simulink model "new_nncACCsystem_4_50"  (R2021a)
(part 10 of 11)

  "IW{4,3}(50,:)'" : Constant  Value=[-0.68975039419682138142064786734408698976039886474609375;-0.337703855474782710377468220031005330383777618408203125;-0.221193087362799634121302005951292812824249267578125;-0.413240348725000650187411110891844145953655242919921875;0.7056367750395093896287335155648179352283477783203125;-0.8247240414571177513636257572215981781482696533203125;-0.368456059408796943177577531969291158020496368408203125;-0.1846558397734467948936298853368498384952545166015625;0.0934305421607941610773195861838757991790771484375;-0.034656334463735671835848961563897319138050079345703125;-0.0169908156708868281203894667896747705526649951934814453125;-0.2111294128865961738927836677248706109821796417236328125;-0.03301633733253335478696754989869077689945697784423828125;-0.453089555771492513702725091206957586109638214111328125;0.90942800382245103651968065605615265667438507080078125;0.784331063728789690259191047516651451587677001953125;-0.0022926906763267584921095476602204144001007080078125;-0.307120717402806775453427690081298351287841796875;0.3730766917773566948568486623116768896579742431640625;0.42980367039944067375500935668242163956165313720703125;-0.12049576378110614383043497355174622498452663421630859375;-0.4758132002910449021015892867580987513065338134765625;-0.86012741082964183636505595131893642246723175048828125;0.7717364942113531522949188001803122460842132568359375;0.4831846028324913167040222106152214109897613525390625;-0.486763294268171275991363700086367316544055938720703125;0.058798309327644800170720174037342076189815998077392578125;0.8066996306207865341519891444477252662181854248046875;-0.69255381214840194825654862142982892692089080810546875;0.1574299186005535811094802056686603464186191558837890625;-0.270336303295735158602752790102385915815830230712890625;0.055888155797568561666821551625616848468780517578125;0.94032669226065757062116290398989804089069366455078125;0.8304969527097798565051789410063065588474273681640625;0.4826285624021837694641590132960118353366851806640625;0.747021101342736582040515713742934167385101318359375;0.391904922693947888046039906839723698794841766357421875;0.764349790072494261750080113415606319904327392578125;-0.7526861421599579937691260056453756988048553466796875;0.240398710986991392957179414224810898303985595703125;-0.0888946820176654828316031853319145739078521728515625;-0.95043102468777018732026817815494723618030548095703125;0.607481136103278362980972815421409904956817626953125;0.5162479599471743174632365480647422373294830322265625;-0.6363106814400574240409014237229712307453155517578125;-0.90826116263117118165837382548488676548004150390625;0.0521855822376402489481961310957558453083038330078125;-0.35977935968636831631783934426493942737579345703125;-0.61308326456983974761527633745572529733180999755859375;-0.4875485158677352881539945883559994399547576904296875]
      mask Display: e = 0.06;c1 = [120 150 230]/255;c2 = ([120 150 230]+0)/383;c3 = ([120 150 230]+128)/383;patch([0 1 1 0],[0 0 1 1],c1);patch([0 1 1 1-e 1-e 0+e],[0 0 1 1-e 0+e 0+e],c2);patch([0 0 1 1-e 0+e 0+e],[0 1 1 1-e 1-e 0+e],c3);plot([0 1 1 0 0],[0 0 1 1 0]);disp('weights');
  "IW{4,3}(6,:)'" : Constant  Value=[0.3760934772975199624767128625535406172275543212890625;0.83188378952229680152186119812540709972381591796875;0.21646625261934016037912442698143422603607177734375;0.4175166061785808846451573117519728839397430419921875;0.245071136922079713116318089305423200130462646484375;-0.2968621138896334610279836851987056434154510498046875;-0.952473185116357701218703368795104324817657470703125;-0.2791944329040980665723736819927580654621124267578125;0.9561025717111750754639842853066511452198028564453125;-0.5509567477390866496733679014141671359539031982421875;0.191023007401977196195730357430875301361083984375;-0.6712729624144617712744320670026354491710662841796875;0.293846976010136540224948475952260196208953857421875;0.5376360375443791639327173470519483089447021484375;-0.689068301622072443279876097221858799457550048828125;-0.9420681689532297564682039592298679053783416748046875;-0.9153320513397549262890606769360601902008056640625;0.7080240151346572918811261843075044453144073486328125;-0.345534410238059308539959602057933807373046875;-0.2596236597249992339442314914776943624019622802734375;0.0156286869832829022897158210980705916881561279296875;0.8238046279287318807149631538777612149715423583984375;0.5409551194199606616308528828085400164127349853515625;-0.539752608426157909349285546340979635715484619140625;-0.47908886469649036854434598353691399097442626953125;-0.309505474526706070292902950313873589038848876953125;0.0077398428835653287904960961895994842052459716796875;-0.775756660878660131430706314858980476856231689453125;0.48844455217338822450301449862308800220489501953125;0.3564821650667175934046326801762916147708892822265625;-0.875481475304413780946788392611779272556304931640625;-0.4156409251020398709641767709399573504924774169921875;0.0110057222602060189586836713715456426143646240234375;-0.8698058882352397436221735915751196444034576416015625;0.3406812767959930265959656026097945868968963623046875;0.4584986472564220871817042279872111976146697998046875;0.5278497841276512669850262682302854955196380615234375;-0.6111457754962399402387518421164713799953460693359375;0.6732737919294760065014315841835923492908477783203125;0.33259267094354338922812530654482543468475341796875;-0.262129955270015368995473181712441146373748779296875;0.140717092303284996290813069208525121212005615234375;0.2060885085486192647152847712277434766292572021484375;-0.1796235649662640820878323211218230426311492919921875;0.4438024646861824518140338113880716264247894287109375;-0.62840596751767474614780439878813922405242919921875;0.0965023358081340543179749147384427487850189208984375;-0.056687085267606018845754078938625752925872802734375;-0.0347507703779630361395902582444250583648681640625;-0.5844728297823975626812398331821896135807037353515625]
      mask Display: e = 0.06;c1 = [120 150 230]/255;c2 = ([120 150 230]+0)/383;c3 = ([120 150 230]+128)/383;patch([0 1 1 0],[0 0 1 1],c1);patch([0 1 1 1-e 1-e 0+e],[0 0 1 1-e 0+e 0+e],c2);patch([0 0 1 1-e 0+e 0+e],[0 1 1 1-e 1-e 0+e],c3);plot([0 1 1 0 0],[0 0 1 1 0]);disp('weights');
  "IW{4,3}(7,:)'" : Constant  Value=[0.8403152974258485397029971863958053290843963623046875;-0.2071458617563731452460018545025377534329891204833984375;-0.723618348300131941641666344366967678070068359375;-0.221142697352507633379303797482862137258052825927734375;0.128396382406429532263558712656958959996700286865234375;-0.1519073900361445073059485366684384644031524658203125;0.9312006523396398893765990578685887157917022705078125;-0.1622147733336041230955970604554750025272369384765625;-0.2574608060089185190832949956529773771762847900390625;-0.7602871717810824048200402103248052299022674560546875;-0.674581332874239603114574492792598903179168701171875;0.339430166289895474118765150706167332828044891357421875;-0.051697509834940529038771472869484568946063518524169921875;0.92405403156981236190148365494678728282451629638671875;-0.85714465050820354274918599912780337035655975341796875;-0.7299230912443717134152620928944088518619537353515625;0.5437820509629733845002874659257940948009490966796875;-0.15716114414254267472870196797885000705718994140625;0.343336796613522399201912094213184900581836700439453125;0.85244575266534761137648956719203852117061614990234375;-0.366396803935940429397533080191351473331451416015625;-0.4758893825967518420583246552268974483013153076171875;-0.281940397738466297372639246532344259321689605712890625;0.25070758776880397444841719334363006055355072021484375;-0.9138567005525863873316438912297599017620086669921875;-0.97612403919302159760462700432981364428997039794921875;0.498327283343458493636290995709714479744434356689453125;0.54675754849605573415516346358344890177249908447265625;-0.81192472217370215137322020382271148264408111572265625;0.7166593175219968525624381072702817618846893310546875;-0.4585059146709802302410707852686755359172821044921875;-0.6980232397374750430429912739782594144344329833984375;-0.7518397450349640909195159110822714865207672119140625;0.973777211720303181863300778786651790142059326171875;-0.286875771908233101470386827713809907436370849609375;0.577485900634702176148493890650570392608642578125;0.3016639899357438370230966029339469969272613525390625;-0.46914794612984156430002258275635540485382080078125;0.6921957739679298615698144203634001314640045166015625;0.911826429592337728280426745186559855937957763671875;-0.097525671829564064552187119261361658573150634765625;-0.357522559522956251409908645655377767980098724365234375;-0.7465707324766157615414385873009450733661651611328125;0.8102029921478746121721314921160228550434112548828125;0.7027792710522238195380850811488926410675048828125;-0.82556198499486865838292715125135146081447601318359375;-0.5517677957555833234692954647471196949481964111328125;-0.923520812028227222612031255266629159450531005859375;0.69847535958997009064574967851513065397739410400390625;0.219645138083222446478970368843874894082546234130859375]
      mask Display: e = 0.06;c1 = [120 150 230]/255;c2 = ([120 150 230]+0)/383;c3 = ([120 150 230]+128)/383;patch([0 1 1 0],[0 0 1 1],c1);patch([0 1 1 1-e 1-e 0+e],[0 0 1 1-e 0+e 0+e],c2);patch([0 0 1 1-e 0+e 0+e],[0 1 1 1-e 1-e 0+e],c3);plot([0 1 1 0 0],[0 0 1 1 0]);disp('weights');
  "IW{4,3}(8,:)'" : Constant  Value=[-0.116688462945323312425216499832458794116973876953125;-0.44605947992465377893722688895650207996368408203125;-0.99658732093286328534986751037649810314178466796875;-0.4783079385244317638381517099332995712757110595703125;-0.2005728686337964195018912505474872887134552001953125;0.3958930317653159836055465348181314766407012939453125;0.0066115562235269376145652131526730954647064208984375;-0.12976532301678833647429200937040150165557861328125;0.862763084062491802939121043891645967960357666015625;0.7666804068579538000705042577465064823627471923828125;0.2002755332553858291788628775975666940212249755859375;0.3224981613712751826739122407161630690097808837890625;-0.7600989470280747895003514713607728481292724609375;0.71268837011036634265792599762789905071258544921875;0.2693318183489117334517004564986564218997955322265625;-0.0214151734751999445194314830587245523929595947265625;0.6479068856290701727829173250938765704631805419921875;0.9944276360022599181576197224785573780536651611328125;-0.1792349111526914118286413213354535400867462158203125;0.45674222060069258333214747835882008075714111328125;0.7704956869907266803210177386063151061534881591796875;-0.0006436272250007757378398309811018407344818115234375;-0.999483386372119309015715771238319575786590576171875;-0.85831423715791288486798293888568878173828125;0.786250856395209307692084621521644294261932373046875;-0.50744024569466983365373380365781486034393310546875;0.4816054146965200732921630333294160664081573486328125;-0.6902006291492128742248723938246257603168487548828125;0.254298316287407732971814766642637550830841064453125;0.519368061486161547435358443181030452251434326171875;-0.790785644673932086590184553642757236957550048828125;-0.68706590989727001073106293915770947933197021484375;-0.558513508754861387473056311137042939662933349609375;0.851974564750733964757500871201045811176300048828125;-0.35667622767825069018954309285618364810943603515625;-0.41145172263983109672835780656896531581878662109375;-0.6493602201676791363382790223113261163234710693359375;-0.5994916295150145568726429701200686395168304443359375;0.4041599000882392100919560107286088168621063232421875;-0.9586288357621561839749801947618834674358367919921875;-0.4832610329434474660814657909213565289974212646484375;-0.842123864413237388504285263479687273502349853515625;-0.561651447245997470503198201186023652553558349609375;0.9176915198905877257828933579730801284313201904296875;-0.43094663445379222110886985319666564464569091796875;0.714815990308057536140040610916912555694580078125;-0.1655937814369423666249758753110654652118682861328125;0.4845374606734373923444536558235995471477508544921875;0.24719870091719453597534084110520780086517333984375;-0.1506864718307741046743331025936640799045562744140625]
      mask Display: e = 0.06;c1 = [120 150 230]/255;c2 = ([120 150 230]+0)/383;c3 = ([120 150 230]+128)/383;patch([0 1 1 0],[0 0 1 1],c1);patch([0 1 1 1-e 1-e 0+e],[0 0 1 1-e 0+e 0+e],c2);patch([0 0 1 1-e 0+e 0+e],[0 1 1 1-e 1-e 0+e],c3);plot([0 1 1 0 0],[0 0 1 1 0]);disp('weights');
  "IW{4,3}(9,:)'" : Constant  Value=[0.954560714917990882355525172897614538669586181640625;0.3907355247891455274356076188269071280956268310546875;0.4785140467488202542511999126872979104518890380859375;-0.376592379022518797260232759072096087038516998291015625;0.893300544264355789181308864499442279338836669921875;-0.193749178232689001077915236237458884716033935546875;-0.46602024758462778919465563376434147357940673828125;-0.2137706950459603572056721532135270535945892333984375;-0.295088615243286778166975636850111186504364013671875;-0.55059251882629689500703307203366421163082122802734375;0.1859857246918747986086373202851973474025726318359375;-0.7383847097081759347503293611225672066211700439453125;0.95986875357167089628518397148582153022289276123046875;-0.54077786815700668032746989410952664911746978759765625;-0.9628262032856012009318646960309706628322601318359375;0.59317539902114280181422145687974989414215087890625;0.58436536663263805024826069711707532405853271484375;-0.5340179474788222524495040488545782864093780517578125;0.75937146836898661295123247327865101397037506103515625;-0.676442785071257102202935129753313958644866943359375;-0.855504824920894524353798260563053190708160400390625;-0.13403199832274792502317950493306852877140045166015625;-0.110797775178757884617652962333522737026214599609375;-0.051205157018530782220278041450001182965934276580810546875;-0.1871836746140778107161395382718183100223541259765625;-0.140905405881837142434420684367069043219089508056640625;-0.783364454271953558617269663955084979534149169921875;0.2111641315298364018904209160609752871096134185791015625;0.910823829267612961047007047454826533794403076171875;0.231589466193370230318038238692679442465305328369140625;0.310157527484731632139158818972646258771419525146484375;0.4978665952885050760556850946159102022647857666015625;-0.387506558926215216587252143654040992259979248046875;0.96150365795292291881679602738586254417896270751953125;-0.094735304889166815911494268220849335193634033203125;0.967857219447221250874235920491628348827362060546875;-0.2322423485804778753305299687781371176242828369140625;0.74864662580344454312353263958357274532318115234375;0.9489155620308868943624247549450956284999847412109375;-0.4060423979950436024211057883803732693195343017578125;0.3119893689463706376585605539730750024318695068359375;0.1879491277425034134740400304508511908352375030517578125;0.93771791705965490404395268342341296374797821044921875;0.4005764539610321417484328776481561362743377685546875;0.35793568702171862927485790351056493818759918212890625;-0.710784392004865761549581293365918099880218505859375;-0.349110480398596489948204180109314620494842529296875;0.0559771506617912084635690916911698877811431884765625;0.07350224902426032158597735133298556320369243621826171875;-0.50203355681308015068253780555096454918384552001953125]
      mask Display: e = 0.06;c1 = [120 150 230]/255;c2 = ([120 150 230]+0)/383;c3 = ([120 150 230]+128)/383;patch([0 1 1 0],[0 0 1 1],c1);patch([0 1 1 1-e 1-e 0+e],[0 0 1 1-e 0+e 0+e],c2);patch([0 0 1 1-e 0+e 0+e],[0 1 1 1-e 1-e 0+e],c3);plot([0 1 1 0 0],[0 0 1 1 0]);disp('weights');
  Mux : Mux  Inputs=50
      mask Display: e = 0.06;c1 = [120 150 230]/255;c2 = ([120 150 230]+0)/383;c3 = ([120 150 230]+128)/383;patch([0 1 1 0],[0 0 1 1],c1);patch([0 1 1 1-e 1-e 0+e],[0 0 1 1-e 0+e 0+e],c2);patch([0 0 1 1-e 0+e 0+e],[0 1 1 1-e 1-e 0+e],c3);plot([0 1 1 0 0],[0 0 1 1 0]);disp('Mux');
  dotprod{1..50} (50 alike) : neural/Weight Functions/dotprod
  "lz{4,3}" : Outport
      mask Display: e = 0.06;c1 = [120 230 180]/255;c2 = ([120 230 180]+0)/(256+128);c3 = ([120 230 180]+128)/(256+128);patch([0 1 1 0],[0 0 1 1],c1);patch([0 1 1 1-e 1-e 0+e],[0 0 1 1-e 0+e 0+e],c2);patch([0 0 1 1-e 0+e 0+e],[0 1 1 1-e 1-e 0+e],c3);plot([0 1 1 0 0],[0 0 1 1 0]);
  wires:
  "IW{4,3}(1,:)'"/1 -> dotprod1/1
  "ad{4,3}"/1 -> dotprod1/2, dotprod2/2, dotprod3/2, dotprod4/2, dotprod5/2, dotprod6/2, dotprod7/2, dotprod8/2, dotprod9/2, dotprod10/2, dotprod11/2, dotprod12/2, dotprod13/2, dotprod14/2, dotprod15/2, dotprod16/2, dotprod17/2, dotprod18/2, dotprod19/2, dotprod20/2, dotprod21/2, dotprod22/2, dotprod23/2, dotprod24/2, dotprod25/2, dotprod26/2, dotprod27/2, dotprod28/2, dotprod29/2, dotprod30/2, dotprod31/2, dotprod32/2, dotprod33/2, dotprod34/2, dotprod35/2, dotprod36/2, dotprod37/2, dotprod38/2, dotprod39/2, dotprod40/2, dotprod41/2, dotprod42/2, dotprod43/2, dotprod44/2, dotprod45/2, dotprod46/2, dotprod47/2, dotprod48/2, dotprod49/2, dotprod50/2
  dotprod1/1 -> Mux/1
  "IW{4,3}(2,:)'"/1 -> dotprod2/1
  dotprod2/1 -> Mux/2
  "IW{4,3}(3,:)'"/1 -> dotprod3/1
  dotprod3/1 -> Mux/3
  "IW{4,3}(4,:)'"/1 -> dotprod4/1
  dotprod4/1 -> Mux/4
  "IW{4,3}(5,:)'"/1 -> dotprod5/1
  dotprod5/1 -> Mux/5
  "IW{4,3}(6,:)'"/1 -> dotprod6/1
  dotprod6/1 -> Mux/6
  "IW{4,3}(7,:)'"/1 -> dotprod7/1
  dotprod7/1 -> Mux/7
  "IW{4,3}(8,:)'"/1 -> dotprod8/1
  dotprod8/1 -> Mux/8
  "IW{4,3}(9,:)'"/1 -> dotprod9/1
  dotprod9/1 -> Mux/9
  "IW{4,3}(10,:)'"/1 -> dotprod10/1
  dotprod10/1 -> Mux/10
  "IW{4,3}(11,:)'"/1 -> dotprod11/1
  dotprod11/1 -> Mux/11
  "IW{4,3}(12,:)'"/1 -> dotprod12/1
  dotprod12/1 -> Mux/12
  "IW{4,3}(13,:)'"/1 -> dotprod13/1
  dotprod13/1 -> Mux/13
  "IW{4,3}(14,:)'"/1 -> dotprod14/1
  dotprod14/1 -> Mux/14
  "IW{4,3}(15,:)'"/1 -> dotprod15/1
  dotprod15/1 -> Mux/15
  "IW{4,3}(16,:)'"/1 -> dotprod16/1
  dotprod16/1 -> Mux/16
  "IW{4,3}(17,:)'"/1 -> dotprod17/1
  dotprod17/1 -> Mux/17
  "IW{4,3}(18,:)'"/1 -> dotprod18/1
  dotprod18/1 -> Mux/18
  "IW{4,3}(19,:)'"/1 -> dotprod19/1
  dotprod19/1 -> Mux/19
  "IW{4,3}(20,:)'"/1 -> dotprod20/1
  dotprod20/1 -> Mux/20
  "IW{4,3}(21,:)'"/1 -> dotprod21/1
  dotprod21/1 -> Mux/21
  "IW{4,3}(22,:)'"/1 -> dotprod22/1
  dotprod22/1 -> Mux/22
  "IW{4,3}(23,:)'"/1 -> dotprod23/1
  dotprod23/1 -> Mux/23
  "IW{4,3}(24,:)'"/1 -> dotprod24/1
  dotprod24/1 -> Mux/24
  "IW{4,3}(25,:)'"/1 -> dotprod25/1
  dotprod25/1 -> Mux/25
  "IW{4,3}(26,:)'"/1 -> dotprod26/1
  dotprod26/1 -> Mux/26
  "IW{4,3}(27,:)'"/1 -> dotprod27/1
  dotprod27/1 -> Mux/27
  "IW{4,3}(28,:)'"/1 -> dotprod28/1
  dotprod28/1 -> Mux/28
  "IW{4,3}(29,:)'"/1 -> dotprod29/1
  dotprod29/1 -> Mux/29
  "IW{4,3}(30,:)'"/1 -> dotprod30/1
  dotprod30/1 -> Mux/30
  "IW{4,3}(31,:)'"/1 -> dotprod31/1
  dotprod31/1 -> Mux/31
  "IW{4,3}(32,:)'"/1 -> dotprod32/1
  dotprod32/1 -> Mux/32
  "IW{4,3}(33,:)'"/1 -> dotprod33/1
  dotprod33/1 -> Mux/33
  "IW{4,3}(34,:)'"/1 -> dotprod34/1
  dotprod34/1 -> Mux/34
  "IW{4,3}(35,:)'"/1 -> dotprod35/1
  dotprod35/1 -> Mux/35
  "IW{4,3}(36,:)'"/1 -> dotprod36/1
  dotprod36/1 -> Mux/36
  "IW{4,3}(37,:)'"/1 -> dotprod37/1
  dotprod37/1 -> Mux/37
  "IW{4,3}(38,:)'"/1 -> dotprod38/1
  dotprod38/1 -> Mux/38
  "IW{4,3}(39,:)'"/1 -> dotprod39/1
  dotprod39/1 -> Mux/39
  "IW{4,3}(40,:)'"/1 -> dotprod40/1
  dotprod40/1 -> Mux/40
  "IW{4,3}(41,:)'"/1 -> dotprod41/1
  dotprod41/1 -> Mux/41
  "IW{4,3}(42,:)'"/1 -> dotprod42/1
  dotprod42/1 -> Mux/42
  "IW{4,3}(43,:)'"/1 -> dotprod43/1
  dotprod43/1 -> Mux/43
  "IW{4,3}(44,:)'"/1 -> dotprod44/1
  dotprod44/1 -> Mux/44
  "IW{4,3}(45,:)'"/1 -> dotprod45/1
  dotprod45/1 -> Mux/45
  "IW{4,3}(46,:)'"/1 -> dotprod46/1
  dotprod46/1 -> Mux/46
  "IW{4,3}(47,:)'"/1 -> dotprod47/1
  dotprod47/1 -> Mux/47
  "IW{4,3}(48,:)'"/1 -> dotprod48/1
  dotprod48/1 -> Mux/48
  "IW{4,3}(49,:)'"/1 -> dotprod49/1
  dotprod49/1 -> Mux/49
  "IW{4,3}(50,:)'"/1 -> dotprod50/1
  dotprod50/1 -> Mux/50
  Mux/1 -> "lz{4,3}"/1
